simulink model "test_seance4_2sorties"  (R2013b)
settings: Solver=ode4  StartTime=0.0  StopTime=0.0149  FixedStep=Te  RelTol=1e-3
values from neighbouring files (symbols this model uses):
  Ka = 0.1    [script_2sorties.m]
  Kb = 0.15    [script_2sorties.m]
  Kd = 10    [script_2sorties.m]
  Te = 1e-4    (= 0.0001)    [script_2sorties.m]
settings Model: TunableVars=Ka,Kb,Kd,Te  TunableVarsStorageClass=Auto,Auto,Auto,Auto  TunableVarsTypeQualifier=,,,  Creator=gemsdev  LastModifiedBy=gemsdev
settings OptimizationCC: InlineParams=on  OptimizeModelRefInitCode=on  LifeSpan=1
settings RTWCC: SystemTargetFile=ert.tlc  TemplateMakefile=RTW.MSVCBuild  Description=Create Visual C/C++ Solution File for Embedded Coder  ProcessScript=ert_make_rtw_hook  TargetLang=C++
settings CodeAppCC: IgnoreCustomStorageClasses=off
settings ERTTargetCC: CodeReplacementLibrary=ANSI_C  GenerateSampleERTMain=on  InlinedParameterPlacement=NonHierarchical  ERTCustomFileTemplate=example_file_process.tlc

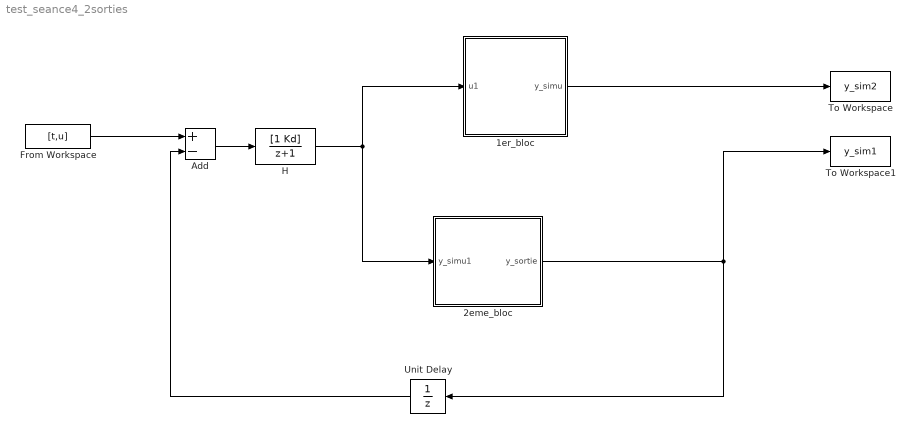
== system test_seance4_2sorties ==
  1er_bloc : Subsystem
  2eme_bloc : Subsystem
  Add : Sum  Inputs=+-
  From Workspace : FromWorkspace  VariableName=[t,u]  SampleTime=0
  H : DiscreteTransferFcn  Numerator=[1 Kd]  Denominator=[1 1]  SampleTime=Te
  To Workspace : ToWorkspace  VariableName=y_sim2  SampleTime=-1
  To Workspace1 : ToWorkspace  VariableName=y_sim1  SampleTime=-1
  Unit Delay : UnitDelay  SampleTime=-1
  wires:
  2eme_bloc/1(y_sortie) -> To Workspace1/1, Unit Delay/1
  From Workspace/1 -> Add/1
  Add/1 -> H/1
  Unit Delay/1 -> Add/2
  H/1 -> 1er_bloc/1(u1), 2eme_bloc/1(y_simu1)
  1er_bloc/1(y_simu) -> To Workspace/1

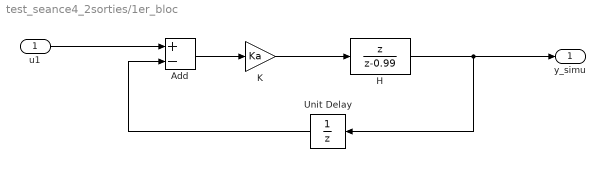
== system test_seance4_2sorties/1er_bloc ==
  u1 : Inport
  Add : Sum  Inputs=+-  SampleTime=Te
  H : DiscreteTransferFcn  Numerator=[1 0]  Denominator=[1 -0.99]  SampleTime=Te
  K : Gain  Gain=Ka  SampleTime=Te
  Unit Delay : UnitDelay  SampleTime=Te
  y_simu : Outport
  wires:
  Add/1 -> K/1
  K/1 -> H/1
  H/1 -> y_simu/1, Unit Delay/1
  Unit Delay/1 -> Add/2
  u1/1 -> Add/1

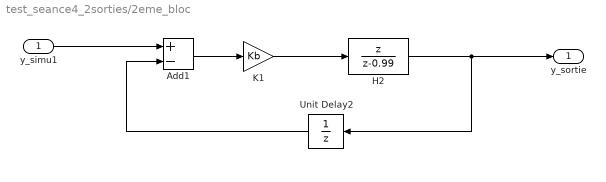
== system test_seance4_2sorties/2eme_bloc ==
  y_simu1 : Inport
  Add1 : Sum  Inputs=+-  SampleTime=Te
  H2 : DiscreteTransferFcn  Numerator=[1 0]  Denominator=[1 -0.99]  SampleTime=Te
  K1 : Gain  Gain=Kb  SampleTime=Te
  Unit Delay2 : UnitDelay  SampleTime=Te
  y_sortie : Outport
  wires:
  y_simu1/1 -> Add1/1
  H2/1 -> y_sortie/1, Unit Delay2/1
  Add1/1 -> K1/1
  Unit Delay2/1 -> Add1/2
  K1/1 -> H2/1
